simulink model "AL_model_PITCH"  (R2023b)
settings: Solver=FixedStepAuto  StartTime=0.0  StopTime=t(end)  FixedStep=t(2)-t(1)  RelTol=1e-3
settings Model: Creator=franc  LastModifiedBy=franc

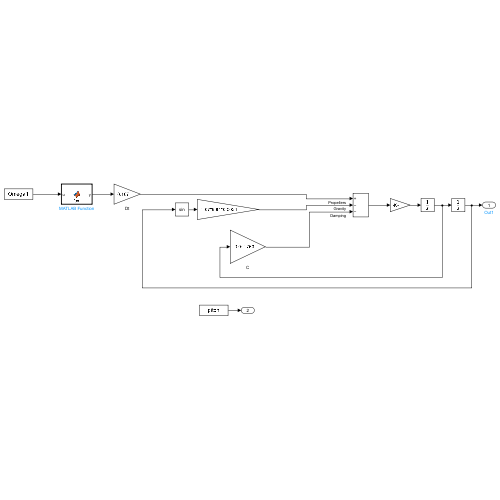
[thumbnail: Simulink's stored preview of the top-level diagram]
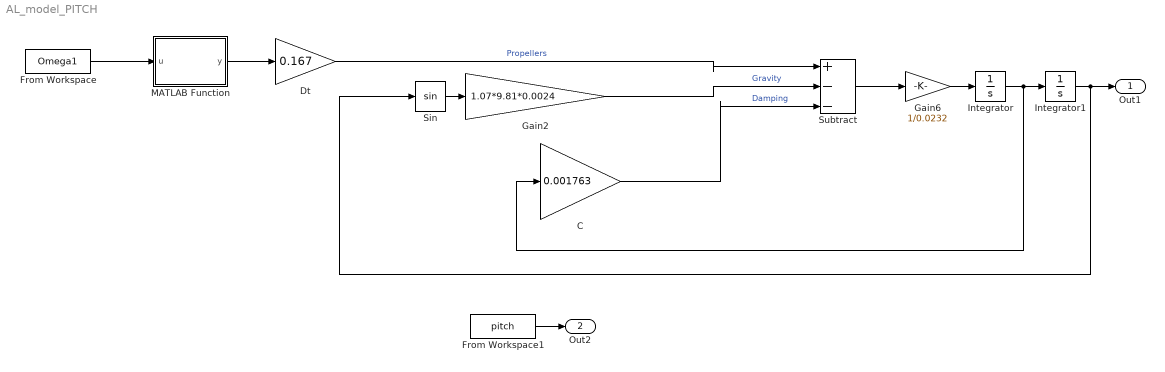
== system AL_model_PITCH ==
  C : Gain  Gain=0.001763
  Dt : Gain  Gain=0.167
  From Workspace : FromWorkspace  VariableName=Omega1  SampleTime=t(2)-t(1)
  From Workspace1 : FromWorkspace  VariableName=pitch
  Gain2 : Gain  Gain=1.07*9.81*0.0024
  Gain6 : Gain  Gain=1/0.0232
  Integrator : Integrator
  Integrator1 : Integrator
  MATLAB Function : MATLAB Function  TreatAsAtomicUnit=on
  Sin : Trigonometry
  Subtract : Sum  Inputs=+--
  Out1 : Outport
  Out2 : Outport  Port=2
  wires:
  Integrator1/1 -> Out1/1, Sin/1
  Dt/1 -> Subtract/1  "Propellers"
  Sin/1 -> Gain2/1
  From Workspace/1 -> MATLAB Function/1(u)
  From Workspace1/1 -> Out2/1
  Gain6/1 -> Integrator/1
  MATLAB Function/1(y) -> Dt/1
  C/1 -> Subtract/3  "Damping"
  Gain2/1 -> Subtract/2  "Gravity"
  Integrator/1 -> Integrator1/1, C/1
  Subtract/1 -> Gain6/1

== matlab function AL_model_PITCH/MATLAB Function ==
  data: u input; y output
function y = fcn(u)

y =-0.00002522922*u+0.00000401487*u^2;
